simulink model "copy2"  (R2021a)
settings: Solver=VariableStepAuto  StartTime=0.0  StopTime=10.0  RelTol=1e-3
libraries: spsSeriesRLCBranchLib x11, spsCurrentMeasurementLib x10, spsVoltageMeasurementLib x4, spsSampleandHoldLib x3, spsGroundLib x2, spsUniversalBridgeLib x2, spsPVArrayLib x1, spsThreePhaseProgrammableVoltageSourceLib x1, pid_lib x1, spspowerguiLib x1
settings Model: Creator=Dell  LastModifiedBy=Dell
settings SolverCC: ZeroCrossControl=DisableAll

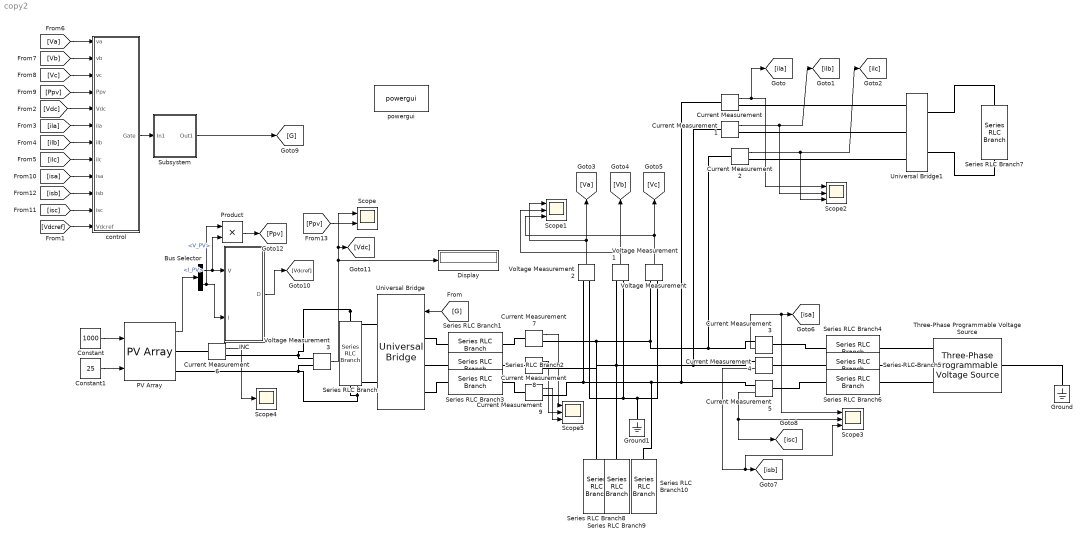
== system copy2 ==
  Bus Selector : BusSelector  OutputSignals=V_PV,I_PV
  Constant : Constant  Value=1000
  Constant1 : Constant  Value=25
  Current Measurement{,1..9} (10 alike) : spsCurrentMeasurementLib/Current Measurement  PhasorSimulation=off  OutputType=Complex  PSBequivalent=0
  Display : Display
  Ground : spsGroundLib/Ground  LConnTagsString=a
  Ground1 : spsGroundLib/Ground  LConnTagsString=a
  INC : Subsystem
  PV Array : spsPVArrayLib/PV Array  Npar=3  Nser=25  PlotType=array @ 1000 W/m2 & specified temperatures  S_vec="[ 1000  500  100 ]"  Temp_C_vec="[ 45 25  ]"  ModuleName=User-defined  PlotWhenSelected=off  Pm=209.175  Ncell=54  Voc=32.8  Isc=8.2  Vm=27.89  Im=7.5  beta_Voc_pc=-0.25  alpha_Isc_pc=0.0031  beta_Voc=-0.082  alpha_Isc=0.0002542  IL=8.2189  I0=2.6394e-12  nI=0.82351  Rsh=70.3148  Rs=0.16177  RobustModel=off  RobustCellTemperature=313.3991  BAL=on  Tc=1e-6  Tfilter=5e-5
  Product : Product
  Scope : Scope  NumInputPorts=2
  Scope{1..3,5} (4 alike) : Scope  NumInputPorts=3
  Scope4 : Scope
  Series RLC Branch : spsSeriesRLCBranchLib/Series RLC Branch  LConnTagsString=__new0  RConnTagsString=__new0  BranchType=C  Resistance=1  Inductance=1e-3  SetiL0=off  InitialCurrent=0  Capacitance=1e-6  Setx0=off  InitialVoltage=0  Measurements=None
  Series RLC Branch1 : spsSeriesRLCBranchLib/Series RLC Branch  LConnTagsString=__new0  RConnTagsString=__new0  BranchType=RL  Resistance=0.272  Inductance=2.5e-3  SetiL0=off  InitialCurrent=0  Capacitance=1e-6  Setx0=off  InitialVoltage=0  Measurements=None
  Series RLC Branch10 : spsSeriesRLCBranchLib/Series RLC Branch  LConnTagsString=__new0  RConnTagsString=__new0  BranchType=RC  Resistance=5  Inductance=1e-3  SetiL0=off  InitialCurrent=0  Capacitance=5e-6  Setx0=off  InitialVoltage=0  Measurements=None
  Series RLC Branch2 : spsSeriesRLCBranchLib/Series RLC Branch  LConnTagsString=__new0  RConnTagsString=__new0  BranchType=RL  Resistance=0.272  Inductance=2.5e-3  SetiL0=off  InitialCurrent=0  Capacitance=1e-6  Setx0=off  InitialVoltage=0  Measurements=None
  Series RLC Branch3 : spsSeriesRLCBranchLib/Series RLC Branch  LConnTagsString=__new0  RConnTagsString=__new0  BranchType=RL  Resistance=0.272  Inductance=2.5e-3  SetiL0=off  InitialCurrent=0  Capacitance=1e-6  Setx0=off  InitialVoltage=0  Measurements=None
  Series RLC Branch4 : spsSeriesRLCBranchLib/Series RLC Branch  LConnTagsString=__new0  RConnTagsString=__new0  BranchType=L  Resistance=0.272  Inductance=3.5e-3  SetiL0=off  InitialCurrent=0  Capacitance=1e-6  Setx0=off  InitialVoltage=0  Measurements=None
  Series RLC Branch5 : spsSeriesRLCBranchLib/Series RLC Branch  LConnTagsString=__new0  RConnTagsString=__new0  BranchType=L  Resistance=0.272  Inductance=3.5e-3  SetiL0=off  InitialCurrent=0  Capacitance=1e-6  Setx0=off  InitialVoltage=0  Measurements=None
  Series RLC Branch6 : spsSeriesRLCBranchLib/Series RLC Branch  LConnTagsString=__new0  RConnTagsString=__new0  BranchType=L  Resistance=0.272  Inductance=3.5e-3  SetiL0=off  InitialCurrent=0  Capacitance=1e-6  Setx0=off  InitialVoltage=0  Measurements=None
  Series RLC Branch7 : spsSeriesRLCBranchLib/Series RLC Branch  LConnTagsString=__new0  RConnTagsString=__new0  BranchType=RL  Resistance=1  Inductance=1e-3  SetiL0=off  InitialCurrent=0  Capacitance=1e-6  Setx0=off  InitialVoltage=0  Measurements=None
  Series RLC Branch8 : spsSeriesRLCBranchLib/Series RLC Branch  LConnTagsString=__new0  RConnTagsString=__new0  BranchType=RC  Resistance=5  Inductance=1e-3  SetiL0=off  InitialCurrent=0  Capacitance=5e-6  Setx0=off  InitialVoltage=0  Measurements=None
  Series RLC Branch9 : spsSeriesRLCBranchLib/Series RLC Branch  LConnTagsString=__new0  RConnTagsString=__new0  BranchType=RC  Resistance=5  Inductance=1e-3  SetiL0=off  InitialCurrent=0  Capacitance=5e-6  Setx0=off  InitialVoltage=0  Measurements=None
  Subsystem : Subsystem
  Three-Phase Programmable Voltage Source : spsThreePhaseProgrammableVoltageSourceLib/Three-Phase Programmable Voltage Source  PositiveSequence="[415  0 50]"  VariationEntity=None  VariationType=Table of time-amplitude pairs  VariationTypeAlt=Step  VariationStep=0.5  VariationRate=10  VariationMagnitude=0.3  VariationFrequency=2  VariationTiming=[1 2]  VariationPhaseA=off  Amplitudes=[1 0.8 1.2 1.0]  TimeValues=[0 0.1 0.15 0.2]  HarmonicGeneration=off  HarmonicA=[3 0.2 -25 0]  HarmonicB=[2 0.15 35 2]  Timing="[0.05  3]"  BusType=swing  Pref=0  Qref=0  Qmin=-inf  Qmax=inf
  Universal Bridge : spsUniversalBridgeLib/Universal Bridge  Arms=3  SnubberResistance=1e5  SnubberCapacitance=inf  Device=IGBT / Diodes  Ron=1e-3  Lon=0  ForwardVoltages="[  0  0  ]"  ForwardVoltage=0  GTOparameters=[ 10e-6 , 20e-6 ]  IGBTparameters=[ 1e-6 , 2e-6 ]  Measurements=None  Measurements_2=None  converterType=Rectifier
  Universal Bridge1 : spsUniversalBridgeLib/Universal Bridge  Arms=3  SnubberResistance=1e5  SnubberCapacitance=inf  Device=Diodes  Ron=1e-3  Lon=0  ForwardVoltages="[  0  0  ]"  ForwardVoltage=0  GTOparameters=[ 10e-6 , 20e-6 ]  IGBTparameters=[ 1e-6 , 2e-6 ]  Measurements=None  Measurements_2=None  converterType=Rectifier
  Voltage Measurement{,1..3} (4 alike) : spsVoltageMeasurementLib/Voltage Measurement  PhasorSimulation=off  OutputType=Complex  PSBequivalent=0
  control : Subsystem
  powergui : spspowerguiLib/powergui  Priority=1  SimulationMode=Continuous  SampleTime=0.001  frequency=60  Iterations=50  frequencyindice=50  Pbase=100e6  ErrMax=1e-4  UnitsV=kV  UnitsW=MW  buscounter=0  FunctionMessages=off  echomessages=off  EnableUseOfTLC=off  CurrentSourceSwitches=off  DisableSnubberDevices=off  DisableRonSwitches=off  DisableVfSwitches=off  DisplayEquations=off  AutomaticDiscreteSolvers=off  SolverType=Tustin/Backward Euler (TBE)  Interpol=off  ExternalGateDelay=off  methode=off  Ts=100  x0status=blocks  SPID=on  SwTol=0  HookPort=off  NonlinearTolerance=1e-4  nMaxIteration=100  ContinueOnMaxIteration=off  RestoreLinks=warning  ResistiveCurrentMeasurement=off  Frange=[0:2:500]  Ylog=off  Xlog=on  ShowGrid=off  save=off  variable=ZData  structure=0  ZoomFFT=off  StartTime=0.0  cycles=1  DisplayStyle=1  fundamental=60  FreqAxis=off  MaxFrequency=1000  frequencyindicesteady=1  RmsSteady=1  display=off
  wires:
  Current Measurement6/1 -> Scope4/1
  [Ppv] -> Scope/2
  Product/1 -> [Ppv]
  [ila] -> control/6(ila)
  Current Measurement3/1 -> Scope3/1, [isa]
  [Vdc] -> control/5(Vdc)
  [Vdcref] -> control/12(Vdcref)
  [ilb] -> control/7(ilb)
  Voltage Measurement3/1 -> Display/1, [Vdc], Scope/1
  [Vb] -> control/2(vb)
  Current Measurement4/1 -> Scope3/3, [isb]
  INC/1(D) -> [Vdcref]
  [G] -> Universal Bridge/1
  Voltage Measurement1/1 -> Scope1/2, [Vb]
  PV Array/1 -> Bus Selector/1
  Voltage Measurement/1 -> Scope1/3, [Vc]
  Voltage Measurement2/1 -> Scope1/1, [Va]
  [isb] -> control/10(isb)
  Subsystem/1(Out1) -> [G]
  Constant/1 -> PV Array/1
  Bus Selector/1 -> Product/2, INC/1(V)  "<V_PV>"
  Current Measurement5/1 -> Scope3/2, [isc]
  [Ppv] -> control/4(Ppv)
  Current Measurement2/1 -> Scope2/3, [ilc]
  [isa] -> control/9(isa)
  [Va] -> control/1(va)
  Current Measurement/1 -> [ila], Scope2/1
  [Vc] -> control/3(vc)
  Current Measurement7/1 -> Scope5/1
  [ilc] -> control/8(ilc)
  control/1(Gate) -> Subsystem/1(In1)
  Current Measurement1/1 -> Scope2/2, [ilb]
  Constant1/1 -> PV Array/2
  Current Measurement9/1 -> Scope5/3
  [isc] -> control/11(isc)
  Current Measurement8/1 -> Scope5/2
  Bus Selector/2 -> Product/1, INC/2(I)  "<I_PV>"
  connections:
  Voltage Measurement2/LConn1 -- Current Measurement9/RConn1 -- Current Measurement/LConn1 -- Current Measurement5/RConn1 -- Series RLC Branch10/RConn1
  Voltage Measurement1/LConn2 -- Voltage Measurement2/LConn2 -- Voltage Measurement/LConn2 -- Ground1/LConn1
  Universal Bridge/RConn2 -- Series RLC Branch/RConn1 -- PV Array/RConn2 -- Voltage Measurement3/LConn2
  Universal Bridge/RConn1 -- Voltage Measurement3/LConn1 -- Current Measurement6/RConn1 -- Series RLC Branch/LConn1
  Current Measurement7/RConn1 -- Series RLC Branch8/RConn1 -- Current Measurement2/LConn1 -- Current Measurement3/RConn1 -- Voltage Measurement/LConn1
  Current Measurement4/RConn1 -- Current Measurement1/LConn1 -- Series RLC Branch9/RConn1 -- Current Measurement8/RConn1 -- Voltage Measurement1/LConn1
  Universal Bridge1/LConn3 -- Current Measurement/RConn1
  Series RLC Branch6/LConn1 -- Current Measurement5/LConn1
  Three-Phase Programmable Voltage Source/RConn1 -- Series RLC Branch4/RConn1
  PV Array/RConn1 -- Current Measurement6/LConn1
  Series RLC Branch5/LConn1 -- Current Measurement4/LConn1
  Series RLC Branch4/LConn1 -- Current Measurement3/LConn1
  Ground/LConn1 -- Three-Phase Programmable Voltage Source/LConn1
  Series RLC Branch2/LConn1 -- Universal Bridge/LConn2
  Universal Bridge1/RConn2 -- Series RLC Branch7/RConn1
  Series RLC Branch3/LConn1 -- Universal Bridge/LConn3
  Three-Phase Programmable Voltage Source/RConn2 -- Series RLC Branch5/RConn1
  Universal Bridge1/LConn2 -- Current Measurement1/RConn1
  Series RLC Branch1/LConn1 -- Universal Bridge/LConn1
  Current Measurement7/LConn1 -- Series RLC Branch1/RConn1
  Three-Phase Programmable Voltage Source/RConn3 -- Series RLC Branch6/RConn1
  Current Measurement9/LConn1 -- Series RLC Branch3/RConn1
  Current Measurement8/LConn1 -- Series RLC Branch2/RConn1
  Universal Bridge1/RConn1 -- Series RLC Branch7/LConn1
  Universal Bridge1/LConn1 -- Current Measurement2/RConn1

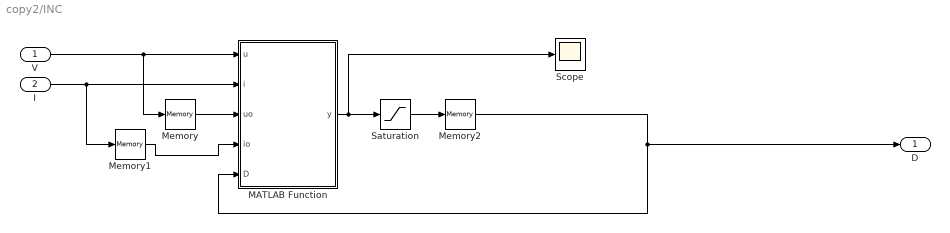
== system copy2/INC ==
  V : Inport
  I : Inport  Port=2
  MATLAB Function : MATLAB Function  TreatAsAtomicUnit=on
  Memory : Memory  InheritSampleTime=on
  Memory1 : Memory  InheritSampleTime=on
  Memory2 : Memory  InheritSampleTime=on
  Saturation : Saturate  UpperLimit=0.9  LowerLimit=0
  Scope : Scope
  D : Outport
  wires:
  Memory/1 -> MATLAB Function/3(uo)
  Saturation/1 -> Memory2/1
  V/1 -> Memory/1, MATLAB Function/1(u)
  Memory1/1 -> MATLAB Function/4(io)
  I/1 -> Memory1/1, MATLAB Function/2(i)
  Memory2/1 -> D/1, MATLAB Function/5(D)
  MATLAB Function/1(y) -> Scope/1, Saturation/1

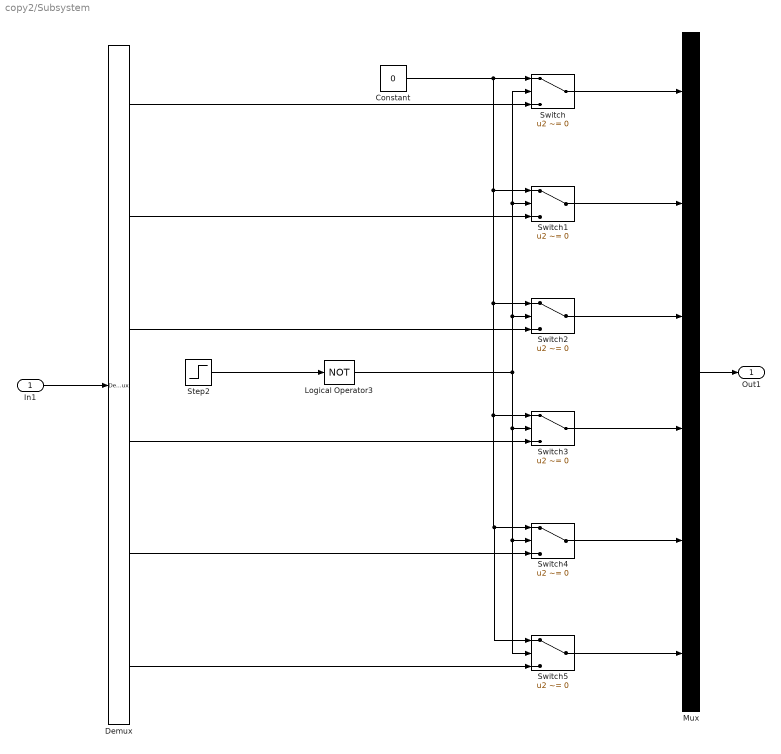
== system copy2/Subsystem ==
  In1 : Inport
  Constant : Constant  Value=0
  Demux : Demux  Outputs=6
  Logical Operator3 : Logic  Operator=NOT  AllPortsSameDT=off  OutDataTypeStr=boolean
  Mux : Mux  Inputs=6
  Step2 : Step  Time=.6  SampleTime=0
  Switch{,1..5} (6 alike) : Switch  Criteria=u2 ~= 0
  Out1 : Outport
  wires:
  Logical Operator3/1 -> Switch3/2, Switch5/2, Switch4/2, Switch/2, Switch1/2, Switch2/2
  Demux/3 -> Switch2/3
  Switch5/1 -> Mux/6
  Switch3/1 -> Mux/4
  Step2/1 -> Logical Operator3/1
  Demux/2 -> Switch1/3
  Demux/6 -> Switch5/3
  Demux/1 -> Switch/3
  Demux/4 -> Switch3/3
  Switch/1 -> Mux/1
  Switch2/1 -> Mux/3
  Demux/5 -> Switch4/3
  Switch1/1 -> Mux/2
  Switch4/1 -> Mux/5
  Constant/1 -> Switch1/1, Switch2/1, Switch5/1, Switch4/1, Switch3/1, Switch/1
  Mux/1 -> Out1/1
  In1/1 -> Demux/1

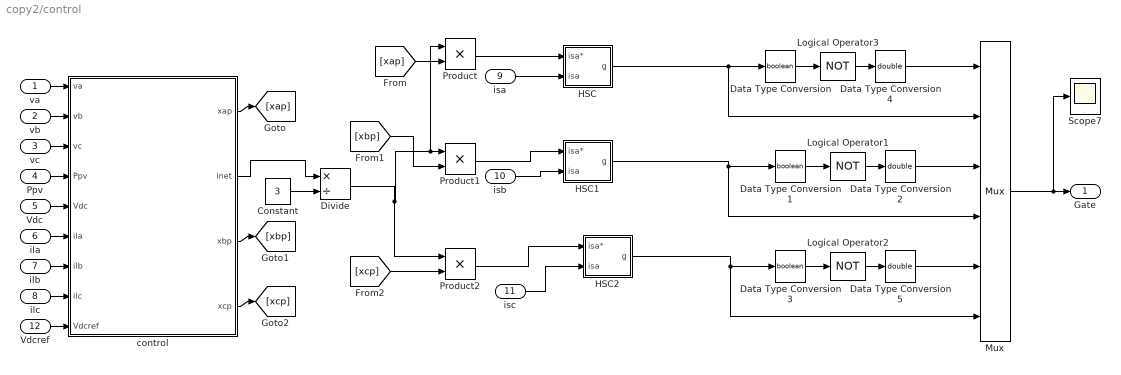
== system copy2/control ==
  va : Inport
  vb : Inport  Port=2
  vc : Inport  Port=3
  Ppv : Inport  Port=4
  Vdc : Inport  Port=5
  ila : Inport  Port=6
  ilb : Inport  Port=7
  ilc : Inport  Port=8
  isa : Inport  Port=9
  isb : Inport  Port=10
  isc : Inport  Port=11
  Vdcref : Inport  Port=12
  Constant : Constant  Value=3
  Data Type Conversion : DataTypeConversion  OutDataTypeStr=boolean  SaturateOnIntegerOverflow=on  RndMeth=Zero
  Data Type Conversion1 : DataTypeConversion  OutDataTypeStr=boolean  SaturateOnIntegerOverflow=on  RndMeth=Zero
  Data Type Conversion2 : DataTypeConversion  OutDataTypeStr=double  SaturateOnIntegerOverflow=on  RndMeth=Zero
  Data Type Conversion3 : DataTypeConversion  OutDataTypeStr=boolean  SaturateOnIntegerOverflow=on  RndMeth=Zero
  Data Type Conversion4 : DataTypeConversion  OutDataTypeStr=double  SaturateOnIntegerOverflow=on  RndMeth=Zero
  Data Type Conversion5 : DataTypeConversion  OutDataTypeStr=double  SaturateOnIntegerOverflow=on  RndMeth=Zero
  Divide : Product  Inputs=*/
  HSC : Subsystem  mask{h=.1}
      mask prompts: h "Hysteresis band (A)"
      mask help: Hysteresis Current Controller
      mask Display: plot(0,0,100,100,[45,45],[35,65],[55,55],[35,65],[45,65],[65,65],[35,55],[35,35])
  HSC1 : Subsystem  mask{h=.1}
      mask prompts: h "Hysteresis band (A)"
      mask help: Hysteresis Current Controller
      mask Display: plot(0,0,100,100,[45,45],[35,65],[55,55],[35,65],[45,65],[65,65],[35,55],[35,35])
  HSC2 : Subsystem  mask{h=.1}
      mask prompts: h "Hysteresis band (A)"
      mask help: Hysteresis Current Controller
      mask Display: plot(0,0,100,100,[45,45],[35,65],[55,55],[35,65],[45,65],[65,65],[35,55],[35,35])
  Logical Operator1 : Logic  Operator=NOT  AllPortsSameDT=off  OutDataTypeStr=boolean
  Logical Operator2 : Logic  Operator=NOT  AllPortsSameDT=off  OutDataTypeStr=boolean
  Logical Operator3 : Logic  Operator=NOT  AllPortsSameDT=off  OutDataTypeStr=boolean
  Mux : Mux  Inputs=6
  Product : Product
  Product1 : Product
  Product2 : Product
  Scope7 : Scope
  control : Subsystem
  Gate : Outport
  wires:
  Product/1 -> HSC/1(isa*)
  Constant/1 -> Divide/2
  Divide/1 -> Product2/1, Product1/1, Product/1
  Product2/1 -> HSC2/1(isa*)
  [xcp] -> Product2/2
  isa/1 -> HSC/2(isa)
  Product1/1 -> HSC1/1(isa*)
  [xbp] -> Product1/2
  control/2(inet) -> Divide/1
  Logical Operator1/1 -> Data Type Conversion2/1
  HSC2/1(g) -> Mux/6, Data Type Conversion3/1
  Data Type Conversion4/1 -> Mux/1
  HSC1/1(g) -> Mux/4, Data Type Conversion1/1
  Data Type Conversion1/1 -> Logical Operator1/1
  Data Type Conversion5/1 -> Mux/5
  Data Type Conversion3/1 -> Logical Operator2/1
  Mux/1 -> Gate/1, Scope7/1
  HSC/1(g) -> Mux/2, Data Type Conversion/1
  Data Type Conversion/1 -> Logical Operator3/1
  Data Type Conversion2/1 -> Mux/3
  Logical Operator2/1 -> Data Type Conversion5/1
  Logical Operator3/1 -> Data Type Conversion4/1
  control/1(xap) -> [xap]
  [xap] -> Product/2
  control/3(xbp) -> [xbp]
  control/4(xcp) -> [xcp]
  va/1 -> control/1(va)
  vb/1 -> control/2(vb)
  vc/1 -> control/3(vc)
  Ppv/1 -> control/4(Ppv)
  Vdc/1 -> control/5(Vdc)
  ila/1 -> control/6(ila)
  ilb/1 -> control/7(ilb)
  ilc/1 -> control/8(ilc)
  isb/1 -> HSC1/2(isa)
  isc/1 -> HSC2/2(isa)
  Vdcref/1 -> control/9(Vdcref)

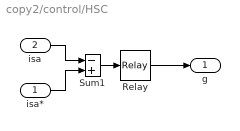
== system copy2/control/HSC ==
  isa* : Inport
  isa : Inport  Port=2
  Relay : Relay  OnSwitchValue=h/2  OffSwitchValue=-h/2
  Sum1 : Sum  Inputs=-+  InputSameDT=on  SaturateOnIntegerOverflow=on  OutDataTypeStr=Inherit: Same as first input
  g : Outport  InitialOutput=0
  wires:
  Sum1/1 -> Relay/1
  Relay/1 -> g/1
  isa/1 -> Sum1/1
  isa*/1 -> Sum1/2

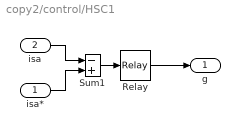
== system copy2/control/HSC1 ==
  isa* : Inport
  isa : Inport  Port=2
  Relay : Relay  OnSwitchValue=h/2  OffSwitchValue=-h/2
  Sum1 : Sum  Inputs=-+  InputSameDT=on  SaturateOnIntegerOverflow=on  OutDataTypeStr=Inherit: Same as first input
  g : Outport  InitialOutput=0
  wires:
  Sum1/1 -> Relay/1
  Relay/1 -> g/1
  isa/1 -> Sum1/1
  isa*/1 -> Sum1/2

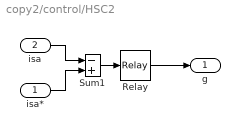
== system copy2/control/HSC2 ==
  isa* : Inport
  isa : Inport  Port=2
  Relay : Relay  OnSwitchValue=h/2  OffSwitchValue=-h/2
  Sum1 : Sum  Inputs=-+  InputSameDT=on  SaturateOnIntegerOverflow=on  OutDataTypeStr=Inherit: Same as first input
  g : Outport  InitialOutput=0
  wires:
  Sum1/1 -> Relay/1
  Relay/1 -> g/1
  isa/1 -> Sum1/1
  isa*/1 -> Sum1/2

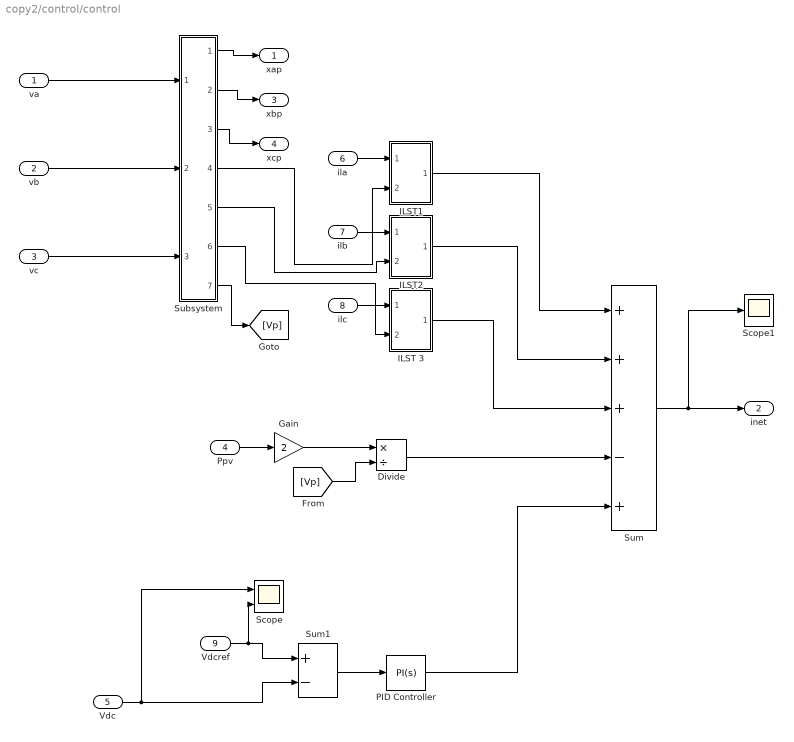
== system copy2/control/control ==
  va : Inport
  vb : Inport  Port=2
  vc : Inport  Port=3
  Ppv : Inport  Port=4
  Vdc : Inport  Port=5
  ila : Inport  Port=6
  ilb : Inport  Port=7
  ilc : Inport  Port=8
  Vdcref : Inport  Port=9
  Divide : Product  Inputs=*/
  Gain : Gain  Gain=2
  ILST 3 : Subsystem
  ILST1 : Subsystem
  ILST2 : Subsystem
  PID Controller : pid_lib/PID Controller  Controller=PI  Form=Parallel  TimeDomain=Continuous-time  UseExternalTs=off  SampleTime=-1  IntegratorMethod=Forward Euler  FilterMethod=Forward Euler  ControllerParametersSource=internal  P=1  I=1  D=0  UseFilter=on  N=100  TunerSelectOption=Transfer Function Based (PID Tuner App)  InitialConditionSource=internal  InitialConditionForIntegrator=0  InitialConditionForFilter=0  DifferentiatorICPrevScaledInput=0  ExternalReset=none  TrackingMode=off  Kt=1  LimitOutput=off  SatLimitsSource=internal  UpperSaturationLimit=inf  LowerSaturationLimit=-inf  LinearizeAsGain=on  AntiWindupMode=none  Kb=1  POutMin=[]  POutMax=[]  IOutMin=[]  IOutMax=[]  DOutMin=[]  DOutMax=[]  NOutMin=[]  NOutMax=[]  SumOutMin=[]  SumOutMax=[]  SaturationOutMin=[]  SaturationOutMax=[]  PParamMin=[]  PParamMax=[]  IParamMin=[]  IParamMax=[]  DParamMin=[]  DParamMax=[]  NParamMin=[]  NParamMax=[]  KbParamMin=[]  KbParamMax=[]  KtParamMin=[]  KtParamMax=[]  KbOutMin=[]  KbOutMax=[]  KtOutMin=[]  KtOutMax=[]  IntegratorOutMin=[]  IntegratorOutMax=[]  FilterOutMin=[]  FilterOutMax=[]  SumI1OutMin=[]  SumI1OutMax=[]  SumI2OutMin=[]  SumI2OutMax=[]  SumI3OutMin=[]  SumI3OutMax=[]  SumI4OutMin=[]  SumI4OutMax=[]  SumDOutMin=[]  SumDOutMax=[]  DifferentiatorOutMin=[]  DifferentiatorOutMax=[]  FilterDiffOutCoefMin=[]  FilterDiffOutCoefMax=[]  ReciprocalOutMin=[]  ReciprocalOutMax=[]  SumDenOutMin=[]  SumDenOutMax=[]  SumNumOutMin=[]  SumNumOutMax=[]  DivideOutMin=[]  DivideOutMax=[]  UdiffTsProdOutMin=[]  UdiffTsProdOutMax=[]  NTsProdOutMin=[]  NTsProdOutMax=[]  UintegralTsProdOutMin=[]  UintegralTsProdOutMax=[]  UngainTsProdOutMin=[]  UngainTsProdOutMax=[]  IntegratorContinuousStateAttributes=''  IntegratorStateMustResolveToSignalObject=off  IntegratorRTWStateStorageClass=Auto  FilterContinuousStateAttributes=''  FilterStateMustResolveToSignalObject=off  FilterRTWStateStorageClass=Auto  ParallelPVariant=InternalParameters  IdealPVariant=Disabled  IVariant=InternalParameters  DVariant=Disabled  IntegratorVariant=Continuous  SatVariant=Disabled  AWVariant=Passthrough  PCopyVariant=Disabled  TRVariant=Disabled  FdbkBlocksVariant=Forward  IdealPFdbkVariant=Disabled  SatFdbkVariant=Disabled  DerivativeFilterVariant=Disabled  NVariant=Disabled  NCopyVariant=Disabled_SignalSpec  FilterICVariant=Disabled  IntegratorICVariant=InternalICs  ExternalResetVariant=Disabled  TRSumVariant=Passthrough  SumFdbkVariant=Disabled  SumVariant=Sum_PI  TsampFilterVariant=InternalTs  TsampNgainVariant=Passthrough  TsampIntegralVariant=Passthrough  ExternalSaturationOutDataTypeStr=Inherit: Same as second input
  Scope : Scope  NumInputPorts=2
  Scope1 : Scope
  Subsystem : Subsystem
  Sum : Sum  Inputs=+++-+
  Sum1 : Sum  Inputs=+-
  xap : Outport
  inet : Outport  Port=2
  xbp : Outport  Port=3
  xcp : Outport  Port=4
  wires:
  Vdcref/1 -> Scope/2, Sum1/1
  ILST2/1(Out1) -> Sum/2
  Sum1/1 -> PID Controller/1
  Ppv/1 -> Gain/1
  ILST1/1(Out1) -> Sum/1
  ILST 3/1(Out1) -> Sum/3
  Vdc/1 -> Sum1/2, Scope/1
  Divide/1 -> Sum/4
  PID Controller/1 -> Sum/5
  Gain/1 -> Divide/1
  Sum/1 -> Scope1/1, inet/1
  vc/1 -> Subsystem/3(Input2)
  vb/1 -> Subsystem/2(Input1)
  va/1 -> Subsystem/1(Input)
  ila/1 -> ILST1/1(In1)
  Subsystem/2(Out2) -> xbp/1
  Subsystem/1(Out1) -> xap/1
  ilb/1 -> ILST2/1(In1)
  Subsystem/6(Out6) -> ILST 3/2(In2)
  Subsystem/5(Out5) -> ILST2/2(In2)
  ilc/1 -> ILST 3/1(In1)
  Subsystem/3(Out3) -> xcp/1
  Subsystem/4(Out4) -> ILST1/2(In2)
  Subsystem/7(Vp) -> [Vp]
  [Vp] -> Divide/2

== system copy2/control/control/ILST 3 ==
  In1 : Inport
  In2 : Inport  Port=2
  ILST3 : Subsystem
  Out1 : Outport
  wires:
  In1/1 -> ILST3/1(In1)
  In2/1 -> ILST3/2(In2)
  ILST3/1(Out1) -> Out1/1

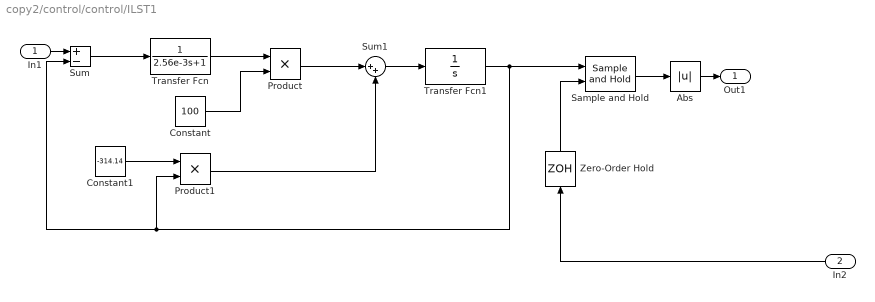
== system copy2/control/control/ILST1 ==
  In1 : Inport
  In2 : Inport  Port=2
  Abs : Abs  ZeroCross=off
  Constant : Constant  Value=100
  Constant1 : Constant  Value=-314.14
  Product : Product
  Product1 : Product
  Sample and Hold : spsSampleandHoldLib/Sample and Hold  ic=0  Ts=0
      settings: SourceProductBaseCode=PS
  Sum : Sum  Inputs=+-
  Sum1 : Sum  Inputs=|++
  Transfer Fcn : TransferFcn  Denominator=[2.56e-3 1]
  Transfer Fcn1 : TransferFcn  Denominator=[1 0]
  Zero-Order Hold : ZeroOrderHold  SampleTime=-1
  Out1 : Outport
  wires:
  Constant/1 -> Product/2
  Constant1/1 -> Product1/1
  Product/1 -> Sum1/1
  Zero-Order Hold/1 -> Sample and Hold/2
  Sum1/1 -> Transfer Fcn1/1
  In1/1 -> Sum/1
  Transfer Fcn1/1 -> Sample and Hold/1, Product1/2, Sum/2
  Product1/1 -> Sum1/2
  Transfer Fcn/1 -> Product/1
  Sum/1 -> Transfer Fcn/1
  Sample and Hold/1 -> Abs/1
  In2/1 -> Zero-Order Hold/1
  Abs/1 -> Out1/1

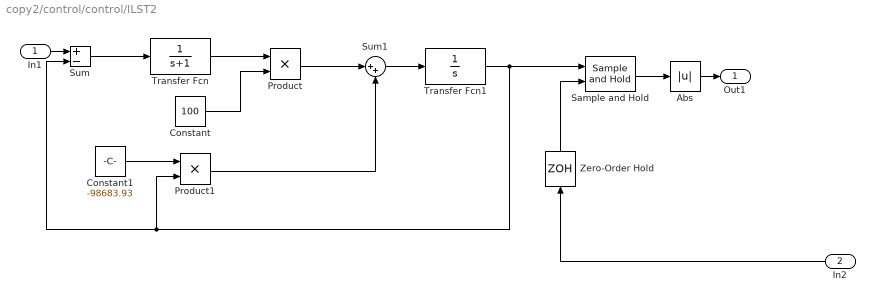
== system copy2/control/control/ILST2 ==
  In1 : Inport
  In2 : Inport  Port=2
  Abs : Abs  ZeroCross=off
  Constant : Constant  Value=100
  Constant1 : Constant  Value=-98683.93
  Product : Product
  Product1 : Product
  Sample and Hold : spsSampleandHoldLib/Sample and Hold  ic=0  Ts=0
      settings: SourceProductBaseCode=PS
  Sum : Sum  Inputs=+-
  Sum1 : Sum  Inputs=|++
  Transfer Fcn : TransferFcn  Denominator=[1 1]
  Transfer Fcn1 : TransferFcn  Denominator=[1 0]
  Zero-Order Hold : ZeroOrderHold  SampleTime=-1
  Out1 : Outport
  wires:
  Constant/1 -> Product/2
  Constant1/1 -> Product1/1
  Product/1 -> Sum1/1
  Zero-Order Hold/1 -> Sample and Hold/2
  Sum1/1 -> Transfer Fcn1/1
  In1/1 -> Sum/1
  Transfer Fcn1/1 -> Sample and Hold/1, Product1/2, Sum/2
  Product1/1 -> Sum1/2
  Transfer Fcn/1 -> Product/1
  Sum/1 -> Transfer Fcn/1
  Sample and Hold/1 -> Abs/1
  In2/1 -> Zero-Order Hold/1
  Abs/1 -> Out1/1

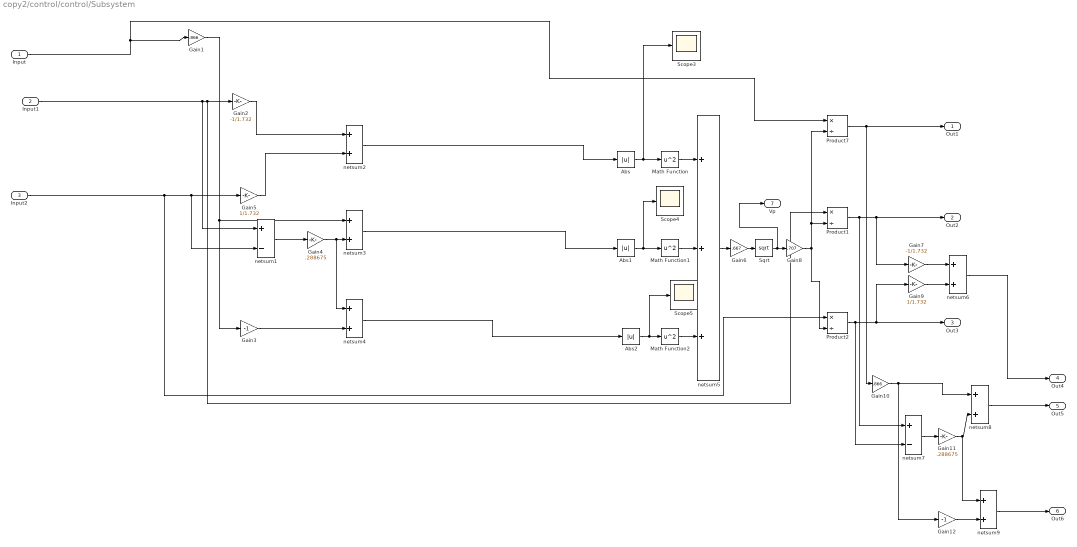
== system copy2/control/control/Subsystem ==
  Input : Inport
  Input1 : Inport  Port=2
  Input2 : Inport  Port=3
  Abs : Abs  ZeroCross=off
  Abs1 : Abs  ZeroCross=off
  Abs2 : Abs  ZeroCross=off
  Gain1 : Gain  Gain=.866
  Gain10 : Gain  Gain=.866
  Gain11 : Gain  Gain=.288675
  Gain12 : Gain  Gain=-1
  Gain2 : Gain  Gain=-1/1.732
  Gain3 : Gain  Gain=-1
  Gain4 : Gain  Gain=.288675
  Gain5 : Gain  Gain=1/1.732
  Gain6 : Gain  Gain=.667
  Gain7 : Gain  Gain=-1/1.732
  Gain8 : Gain  Gain=.707
  Gain9 : Gain  Gain=1/1.732
  Math Function : Math  Operator=square  SignedPower=on  SaturateOnIntegerOverflow=on
  Math Function1 : Math  Operator=square  SignedPower=on  SaturateOnIntegerOverflow=on
  Math Function2 : Math  Operator=square  SignedPower=on  SaturateOnIntegerOverflow=on
  Product1 : Product  Inputs=*/  RndMeth=Zero
  Product2 : Product  Inputs=*/  RndMeth=Zero
  Product7 : Product  Inputs=*/  RndMeth=Zero
  Scope3 : Scope
  Scope4 : Scope
  Scope5 : Scope
  Sqrt : Sqrt  SaturateOnIntegerOverflow=on
  netsum1 : Sum  Inputs=+-  InputSameDT=on  SaturateOnIntegerOverflow=on  OutDataTypeStr=Inherit: Same as first input
  netsum{2..4,6,8..9} (6 alike) : Sum  InputSameDT=on  SaturateOnIntegerOverflow=on  OutDataTypeStr=Inherit: Same as first input
  netsum5 : Sum  Inputs=+++  InputSameDT=on  SaturateOnIntegerOverflow=on  OutDataTypeStr=Inherit: Same as first input
  netsum7 : Sum  Inputs=+-  InputSameDT=on  SaturateOnIntegerOverflow=on  OutDataTypeStr=Inherit: Same as first input
  Out1 : Outport
  Out2 : Outport  Port=2
  Out3 : Outport  Port=3
  Out4 : Outport  Port=4
  Out5 : Outport  Port=5
  Out6 : Outport  Port=6
  Vp : Outport  Port=7
  wires:
  Input2/1 -> Product2/1, netsum1/2, Gain5/1
  Input1/1 -> netsum1/1, Product1/1, Gain2/1
  Gain9/1 -> netsum6/2
  Gain8/1 -> Product2/2, Product7/2, Product1/2
  Gain12/1 -> netsum9/2
  netsum2/1 -> Abs/1
  netsum9/1 -> Out6/1
  Gain3/1 -> netsum4/2
  netsum7/1 -> Gain11/1
  Gain4/1 -> netsum4/1, netsum3/2
  Gain5/1 -> netsum2/2
  netsum1/1 -> Gain4/1
  Math Function2/1 -> netsum5/3
  Gain1/1 -> Gain3/1, netsum3/1
  netsum8/1 -> Out5/1
  Product7/1 -> Gain10/1, Out1/1
  Gain2/1 -> netsum2/1
  Product2/1 -> netsum7/2, Gain9/1, Out3/1
  Math Function/1 -> netsum5/1
  Input/1 -> Product7/1, Gain1/1
  Product1/1 -> netsum7/1, Out2/1, Gain7/1
  netsum3/1 -> Abs1/1
  Sqrt/1 -> Vp/1, Gain8/1
  Abs2/1 -> Scope5/1, Math Function2/1
  Gain11/1 -> netsum9/1, netsum8/2
  Abs1/1 -> Scope4/1, Math Function1/1
  netsum5/1 -> Gain6/1
  Gain6/1 -> Sqrt/1
  Math Function1/1 -> netsum5/2
  netsum4/1 -> Abs2/1
  Gain7/1 -> netsum6/1
  netsum6/1 -> Out4/1
  Gain10/1 -> Gain12/1, netsum8/1
  Abs/1 -> Scope3/1, Math Function/1

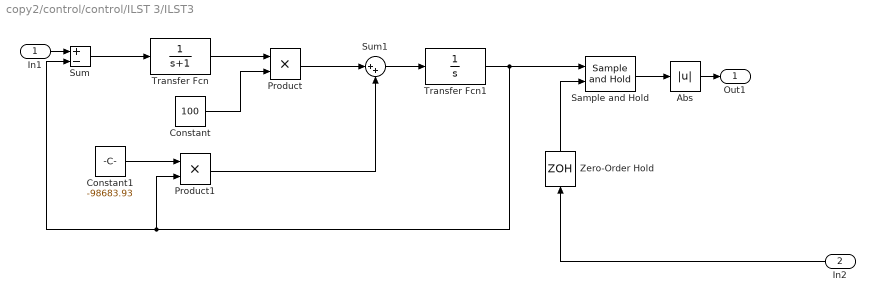
== system copy2/control/control/ILST 3/ILST3 ==
  In1 : Inport
  In2 : Inport  Port=2
  Abs : Abs  ZeroCross=off
  Constant : Constant  Value=100
  Constant1 : Constant  Value=-98683.93
  Product : Product
  Product1 : Product
  Sample and Hold : spsSampleandHoldLib/Sample and Hold  ic=0  Ts=0
      settings: SourceProductBaseCode=PS
  Sum : Sum  Inputs=+-
  Sum1 : Sum  Inputs=|++
  Transfer Fcn : TransferFcn  Denominator=[1 1]
  Transfer Fcn1 : TransferFcn  Denominator=[1 0]
  Zero-Order Hold : ZeroOrderHold  SampleTime=-1
  Out1 : Outport
  wires:
  Constant/1 -> Product/2
  Constant1/1 -> Product1/1
  Product/1 -> Sum1/1
  Zero-Order Hold/1 -> Sample and Hold/2
  Sum1/1 -> Transfer Fcn1/1
  In1/1 -> Sum/1
  Transfer Fcn1/1 -> Sample and Hold/1, Product1/2, Sum/2
  Product1/1 -> Sum1/2
  Transfer Fcn/1 -> Product/1
  Sum/1 -> Transfer Fcn/1
  Sample and Hold/1 -> Abs/1
  In2/1 -> Zero-Order Hold/1
  Abs/1 -> Out1/1

== matlab function copy2/INC/MATLAB Function ==
  data: u input; y output; i input; uo input; io input; D input
function y = MYMPP(u,i,uo,io,D)
m=0.4;
du=u-uo;
di=i-io;
d=0.00005;
if du==0
    if di==0
    m=D;
    else
        if di>0
            m=D-d;
        else
            m=D+d;
        end
    end
else
    if di/du== -(i/u)
    m=D;
    else
        if di/du> -(i/u)
        m=D-d;
        else
            m=D+d;
        end
    end
end
y = m;
end
